simulink model "sim_new_traj_only_pos_ctrl"  (R2020a)
settings: Solver=ode4  StartTime=0.0  StopTime=30.0  FixedStep=0.01  RelTol=1e-3
values from neighbouring files (symbols this model uses):
  alfa_theta = 20    [init_new_traj_only_pos_ctrl.m]
  alfa_theta_obs = 100    [init_new_traj_only_pos_ctrl.m]
  beta1 = 1.2    [init_new_traj_only_pos_ctrl.m]
  beta2 = 0.8    [init_new_traj_only_pos_ctrl.m]
  c1_diff_sigma_bar_v = diag([25; 30; 20])    [init_new_traj_only_pos_ctrl.m]
  c1v = diag([5.8; 6.5; 6.5])    [init_new_traj_only_pos_ctrl.m]
  c2_diff_sigma_bar_v = diag([50; 50; 10])    [init_new_traj_only_pos_ctrl.m]
  c2v = diag([5.8; 6.5; 6.5])    [init_new_traj_only_pos_ctrl.m]
  c3_diff_sigma_bar_v = diag([15; 15; 10])    [init_new_traj_only_pos_ctrl.m]
  c3v = diag([4.8; 6.4; 6.0])    [init_new_traj_only_pos_ctrl.m]
  delta_p_i_0 = zeros(3, NF)    [init_new_traj_only_pos_ctrl.m]
  delta_v_i_0 = zeros(3, NF)    [init_new_traj_only_pos_ctrl.m]
  dp_aa_t = 0.2 * ones(3, 5) + ( 1.0 - 0.2 ) * rand(3, 5)    [init_new_traj_only_pos_ctrl.m]
  dp_ff_t = [ 0.4 * ones(1, 5) + ( 1.0 - 0.4 ) * rand(1, 5);                      0.4 * ones(1, 5) + ( 1.0 - 0.4 ) * rand(1, 5);                      0.2 * ones(1, 5) + ( 0.6 - 0.2 ) * rand(1, 5) ]    [init_new_traj_only_pos_ctrl.m]
  dp_phi_t = ( - pi / 2 ) * ones(3, 5) + ( pi / 2 - ( - pi / 2 ) ) * rand(3, 5)    [init_new_traj_only_pos_ctrl.m]
  etai_0 = zeros(3,5)    [init_new_traj_only_pos_ctrl.m]
  kai_1_t = 0.02    [init_new_traj_only_pos_ctrl.m]
  kai_3_t = 0.1    [init_new_traj_only_pos_ctrl.m]
  kai_chi_1 = diag([6; 6; 6])    [init_new_traj_only_pos_ctrl.m]
  kai_chi_2 = diag([6; 6; 6])    [init_new_traj_only_pos_ctrl.m]
  kai_u_1 = diag([8; 8; 8])    [init_new_traj_only_pos_ctrl.m]
  kai_u_2 = diag([8; 8; 8])    [init_new_traj_only_pos_ctrl.m]
  ksii_0 = zeros(3,5)    [init_new_traj_only_pos_ctrl.m]
  l1v = diag([20; 20; 20])    [init_new_traj_only_pos_ctrl.m]
  l2v = diag([30; 30; 30])    [init_new_traj_only_pos_ctrl.m]
  Lamd_diff_sigma_bar_v = 0.5    [init_new_traj_only_pos_ctrl.m]
  mass_i = zeros(1,NF)    [init_new_traj_only_pos_ctrl.m]
  Mii = diag([1;0;0;0;1])    [init_new_traj_only_pos_ctrl.m]
  pos0 = zeros(3, 1)    [init_new_traj_only_pos_ctrl.m]
  PZ0 = P0(3)    [init_new_traj_only_pos_ctrl.m]
  PZ1 = 10    [init_new_traj_only_pos_ctrl.m]
  Qci_init = repmat([1;0;0;0],1,NF)    [init_new_traj_only_pos_ctrl.m]
  R0 = 4    [init_new_traj_only_pos_ctrl.m]
  R1 = 8    [init_new_traj_only_pos_ctrl.m]
  Rx2 = 10    [init_new_traj_only_pos_ctrl.m]
  Ry2 = 6    [init_new_traj_only_pos_ctrl.m]
  Rz2 = 4    [init_new_traj_only_pos_ctrl.m]
  T0 = 0    [init_new_traj_only_pos_ctrl.m]
  T1 = tseq1    (= 10)    [init_new_traj_only_pos_ctrl.m]
  T12 = tseq1 + tseq12    (= 20)    [init_new_traj_only_pos_ctrl.m]
  T2 = tseq1 + tseq12 + tseq2    (= 30)    [init_new_traj_only_pos_ctrl.m]
  theta0 = ( 2 / 5 ) * pi    (= 1.25663706144)    [init_new_traj_only_pos_ctrl.m]
  vel0 = zeros(3, 1)    [init_new_traj_only_pos_ctrl.m]
  Wij = [0,0,1,0,0;              0,0,1,1,0;              1,0,0,0,1;              0,1,1,0,0;              0,0,1,0,0]    [init_new_traj_only_pos_ctrl.m]
  X1 = 8    [init_new_traj_only_pos_ctrl.m]
  X2 = 2    [init_new_traj_only_pos_ctrl.m]
  X3 = 3    [init_new_traj_only_pos_ctrl.m]
  Y1 = 10    [init_new_traj_only_pos_ctrl.m]
  Y2 = 2    [init_new_traj_only_pos_ctrl.m]
  Y3 = 4    [init_new_traj_only_pos_ctrl.m]
  Z1 = 4    [init_new_traj_only_pos_ctrl.m]
  Z2 = -6    [init_new_traj_only_pos_ctrl.m]
  Z3 = 2    [init_new_traj_only_pos_ctrl.m]
  zeta_diff_sigma_bar_v = 0.08    [init_new_traj_only_pos_ctrl.m]
undefined symbols (not defined in the file or in its folder): cal_frac_squ, p_alfav1, p_alfav2, p_beta1, p_beta2, p_dbeta1, p_dbeta2, p_gamma1_pos, p_gamma1_vel, p_gamma2_pos, p_gamma2_vel, q_alfav1, q_alfav2, q_beta1, q_beta2, q_dbeta1, q_dbeta2, q_gamma1_pos, q_gamma1_vel, q_gamma2_pos, q_gamma2_vel
(part 4 of 5)

== matlab function sim_new_traj_only_pos_ctrl/set desire formation configuration ==
  data: X1 input; X2 input; X3 input; Y1 input; Y2 input; Y3 input; Z1 input; Z2 input; Z3 input; theta0 input; kai_1_t input; kai_3_t input; T1 input; T12 input; t input; delta_ksi_vec output; delta_eta_vec output
function [delta_ksi_vec, delta_eta_vec] = fcn(X1, X2, X3, Y1, Y2, Y3, Z1, Z2, Z3, theta0, ...
                                                                                    kai_1_t, kai_3_t, T1, T12, t)
%%%% 计算跟随者期望速度分布式观测器误差
delta_ksi_vec = zeros(3, 5);
delta_eta_vec = zeros(3, 5);
if t <= ( T1 + 1e-04 )
    exp_tmp = exp( -kai_1_t * t );
    delta_ksi_vec(:, 1) = [ X1 * cos( theta0 ) - X2 * exp_tmp; ...
                                            Y1 * sin( theta0 ) - Y2 * exp_tmp; ...
                                            Z1 - Z2 * exp_tmp ];
    delta_ksi_vec(:, 2) = [ - X1 * cos( theta0 ) + X2 * exp_tmp; ...
                                            Y1 * sin( theta0 ) - Y2 * exp_tmp; ...
                                            Z1 + Z2 * exp_tmp ];
    delta_ksi_vec(:, 3) = [ X1 - X2 * exp_tmp; ...
                                            Y2 * exp_tmp; ...
                                            ( 3 / 8 ) * Z1 + Z2 * exp_tmp ];
    delta_ksi_vec(:, 4) = [ - X1 * cos( theta0 ) + X2 * exp_tmp; ...
                                            - Y1 * sin( theta0 ) + Y2 * exp_tmp; ...
                                            Z1 + Z2 * exp_tmp ];
    delta_ksi_vec(:, 5) = [ X1 * cos( theta0 ) - X2 * exp_tmp; ...
                                            - Y1 * sin( theta0 ) + Y2 * exp_tmp; ...
                                            Z1 - Z2 * exp_tmp ];
    delta_eta_vec(:, 1) = [ kai_1_t * X2 * exp_tmp; kai_1_t * Y2 * exp_tmp; kai_1_t * Z2 * exp_tmp ];
    delta_eta_vec(:, 2) = [ - kai_1_t * X2 * exp_tmp; kai_1_t * Y2 * exp_tmp; - kai_1_t * Z2 * exp_tmp ];
    delta_eta_vec(:, 3) = [ kai_1_t * X2 * exp_tmp; - kai_1_t * Y2 * exp_tmp; - kai_1_t * Z2 * exp_tmp ];
    delta_eta_vec(:, 4) = [ - kai_1_t * X2 * exp_tmp; - kai_1_t * Y2 * exp_tmp; - kai_1_t * Z2 * exp_tmp ];
    delta_eta_vec(:, 5) = [ kai_1_t * X2 * exp_tmp; - kai_1_t * Y2 * exp_tmp; kai_1_t * Z2 * exp_tmp ];
elseif t <= ( T12 + 1e-04 )
    delta_ksi_vec(:, 1) = [ X1 * cos( theta0 ) - X2; Y1 * sin( theta0 ) - Y2; Z1 - Z2 ];
    delta_ksi_vec(:, 2) = [ - X1 * cos( theta0 ) + X2; Y1 * sin( theta0 ) - Y2; Z1 + Z2 ];
    delta_ksi_vec(:, 3) = [ X1 - X2; 0; ( 3 / 8 ) * Z1 + Z2 ];
    delta_ksi_vec(:, 4) = [ - X1 * cos( theta0 ) + X2; - Y1 * sin( theta0 ) + Y2; Z1 + Z2 ];
    delta_ksi_vec(:, 5) = [ X1 * cos( theta0 ) - X2; - Y1 * sin( theta0 ) + Y2; Z1 - Z2 ];
else
    exp_tmp = 1 / ( 1 + exp( - kai_3_t * ( t - T12 - 5 ) ) );
    tmp_2 = exp( - kai_3_t * ( t - T12 - 5 ) ) / ( ( 1 + exp( - kai_3_t * ( t - T12 - 5 ) ) ) ^ 2 );
    delta_ksi_vec(:, 1) = [ X1 * cos( theta0 ) - X2 + X3 * exp_tmp; ...
                                            Y1 * sin( theta0 ) - Y2 + Y3 * exp_tmp; ...
                                            Z1 - Z2 + Z3 * exp_tmp ];
    delta_ksi_vec(:, 2) = [ - X1 * cos( theta0 ) + X2 - X3 * exp_tmp; ...
                                            Y1 * sin( theta0 ) - Y2 + Y3 * exp_tmp; ...
                                            Z1 + Z2 - Z3 * exp_tmp ];
    delta_ksi_vec(:, 3) = [ X1 - X2 + X3 * exp_tmp; ...
                                            - Y3 * exp_tmp; ...
                                            ( 3 / 8 ) * Z1 + Z2 - Z3 * exp_tmp ];
    delta_ksi_vec(:, 4) = [ - X1 * cos( theta0 ) + X2 - X3 * exp_tmp; ...
                                            - Y1 * sin( theta0 ) + Y2 - Y3 * exp_tmp; ...
                                            Z1 + Z2 - Z3 * exp_tmp ];
    delta_ksi_vec(:, 5) = [ X1 * cos( theta0 ) - X2 + X3 * exp_tmp; ...
                                            - Y1 * sin( theta0 ) + Y2 - Y3 * exp_tmp; ...
                                            Z1 - Z2 + Z3 * exp_tmp ];
    delta_eta_vec(:, 1) = [ kai_3_t * X3 * tmp_2; kai_3_t * Y3 * tmp_2; kai_3_t * Z3 * tmp_2 ];
    delta_eta_vec(:, 2) = [ - kai_3_t * X3 * tmp_2; kai_3_t * Y3 * tmp_2; kai_3_t * Z3 * tmp_2 ];
    delta_eta_vec(:, 3) = [ kai_3_t * X3 * tmp_2; - kai_3_t * Y3 * tmp_2; - kai_3_t * Z3 * tmp_2 ];
    delta_eta_vec(:, 4) = [ - kai_3_t * X3 * tmp_2; - kai_3_t * Y3 * tmp_2; - kai_3_t * Z3 * tmp_2 ];
    delta_eta_vec(:, 5) = [ kai_3_t * X3 * tmp_2; kai_3_t * Y3 * tmp_2; - kai_3_t * Z3 * tmp_2 ];
end

== matlab function sim_new_traj_only_pos_ctrl/choose dp_tilt_5 ==
  data: x input; y output
function y = fcn(x)
iiuav = 5;
y = x(:,iiuav);

== matlab function sim_new_traj_only_pos_ctrl/choose sigma_bar_v_tilt_5 ==
  data: x input; y output
function y = fcn(x)
iiuav = 5;
y = x(:,iiuav);

== matlab function sim_new_traj_only_pos_ctrl/choose sigma_bar_v_tilt_1 ==
  data: x input; y output
function y = fcn(x)
iiuav = 1;
y = x(:,iiuav);

== matlab function sim_new_traj_only_pos_ctrl/choose sigma_bar_v_tilt_2 ==
  data: x input; y output
function y = fcn(x)
iiuav = 2;
y = x(:,iiuav);

== matlab function sim_new_traj_only_pos_ctrl/choose sigma_bar_v_tilt_3 ==
  data: x input; y output
function y = fcn(x)
iiuav = 3;
y = x(:,iiuav);

== matlab function sim_new_traj_only_pos_ctrl/choose sigma_bar_v_tilt_4 ==
  data: x input; y output
function y = fcn(x)
iiuav = 4;
y = x(:,iiuav);

== matlab function sim_new_traj_only_pos_ctrl/choose phi_5 ==
  data: x input; y output
function y = fcn(x)
iiuav = 5;
y = x(:,iiuav);

== matlab function sim_new_traj_only_pos_ctrl/choose phi_1 ==
  data: x input; y output
function y = fcn(x)
iiuav = 1;
y = x(:,iiuav);

== matlab function sim_new_traj_only_pos_ctrl/choose phi_2 ==
  data: x input; y output
function y = fcn(x)
iiuav = 2;
y = x(:,iiuav);

== matlab function sim_new_traj_only_pos_ctrl/choose phi_3 ==
  data: x input; y output
function y = fcn(x)
iiuav = 3;
y = x(:,iiuav);

== matlab function sim_new_traj_only_pos_ctrl/choose phi_4 ==
  data: x input; y output
function y = fcn(x)
iiuav = 4;
y = x(:,iiuav);

== matlab function sim_new_traj_only_pos_ctrl/choose err_eta_1 ==
  data: x input; y output
function y = fcn(x)
iiuav = 1;
y = x(:,iiuav);

== matlab function sim_new_traj_only_pos_ctrl/choose chi_1 ==
  data: x input; y output
function y = fcn(x)
iiuav = 1;
y = x(:,iiuav);

== matlab function sim_new_traj_only_pos_ctrl/choose chi_2 ==
  data: x input; y output
function y = fcn(x)
iiuav = 2;
y = x(:,iiuav);

== matlab function sim_new_traj_only_pos_ctrl/choose err_eta_2 ==
  data: x input; y output
function y = fcn(x)
iiuav = 2;
y = x(:,iiuav);

== matlab function sim_new_traj_only_pos_ctrl/choose chi_3 ==
  data: x input; y output
function y = fcn(x)
iiuav = 3;
y = x(:,iiuav);

== matlab function sim_new_traj_only_pos_ctrl/choose err_eta_3 ==
  data: x input; y output
function y = fcn(x)
iiuav = 3;
y = x(:,iiuav);

== matlab function sim_new_traj_only_pos_ctrl/choose chi_4 ==
  data: x input; y output
function y = fcn(x)
iiuav = 4;
y = x(:,iiuav);

== matlab function sim_new_traj_only_pos_ctrl/choose err_eta_4 ==
  data: x input; y output
function y = fcn(x)
iiuav = 4;
y = x(:,iiuav);

== matlab function sim_new_traj_only_pos_ctrl/choose chi_5 ==
  data: x input; y output
function y = fcn(x)
iiuav = 5;
y = x(:,iiuav);

== matlab function sim_new_traj_only_pos_ctrl/choose err_eta_5 ==
  data: x input; y output
function y = fcn(x)
iiuav = 5;
y = x(:,iiuav);

== matlab function sim_new_traj_only_pos_ctrl/choose sigma_bar_v_hat_5 ==
  data: x input; y output
function y = fcn(x)
iiuav = 5;
y = x(:,iiuav);

== matlab function sim_new_traj_only_pos_ctrl/choose sigma_bar_v_hat_1 ==
  data: x input; y output
function y = fcn(x)
iiuav = 1;
y = x(:,iiuav);

== matlab function sim_new_traj_only_pos_ctrl/choose sigma_bar_v_hat_2 ==
  data: x input; y output
function y = fcn(x)
iiuav = 2;
y = x(:,iiuav);

== matlab function sim_new_traj_only_pos_ctrl/choose sigma_bar_v_hat_3 ==
  data: x input; y output
function y = fcn(x)
iiuav = 3;
y = x(:,iiuav);

== matlab function sim_new_traj_only_pos_ctrl/choose sigma_bar_v_hat_4 ==
  data: x input; y output
function y = fcn(x)
iiuav = 4;
y = x(:,iiuav);

== matlab function sim_new_traj_only_pos_ctrl/choose sigma_bar_v_5 ==
  data: x input; y output
function y = fcn(x)
iiuav = 5;
y = x(:,iiuav);

== matlab function sim_new_traj_only_pos_ctrl/choose sigma_bar_v_1 ==
  data: x input; y output
function y = fcn(x)
iiuav = 1;
y = x(:,iiuav);

== matlab function sim_new_traj_only_pos_ctrl/choose sigma_bar_v_2 ==
  data: x input; y output
function y = fcn(x)
iiuav = 2;
y = x(:,iiuav);

== matlab function sim_new_traj_only_pos_ctrl/choose sigma_bar_v_3 ==
  data: x input; y output
function y = fcn(x)
iiuav = 3;
y = x(:,iiuav);

== matlab function sim_new_traj_only_pos_ctrl/choose sigma_bar_v_4 ==
  data: x input; y output
function y = fcn(x)
iiuav = 4;
y = x(:,iiuav);

== matlab function sim_new_traj_only_pos_ctrl/cal formation tracking position and velocity errors ==
  data: ksi_i_vec input; err_ksi_vec output; ksi_d_est_vec input; eta_i_vec input; eta_d_est_vec input; err_eta_vec output
function [err_ksi_vec, err_eta_vec] = fcn(ksi_i_vec, ksi_d_est_vec, eta_i_vec, eta_d_est_vec)
%%%% 计算编队跟踪误差
err_ksi_vec = zeros(3,5);
err_eta_vec = zeros(3,5);
for iiuav = 1:5
    err_ksi_vec(:,iiuav) = ksi_i_vec(:,iiuav) - ksi_d_est_vec(:,iiuav);
    err_eta_vec(:,iiuav) = eta_i_vec(:,iiuav) - eta_d_est_vec(:,iiuav);
end

== matlab function sim_new_traj_only_pos_ctrl/choose dp_5 ==
  data: x input; y output
function y = fcn(x)
iiuav = 5;
y = x(:,iiuav);

== matlab function sim_new_traj_only_pos_ctrl/choose dp_1 ==
  data: x input; y output
function y = fcn(x)
iiuav = 1;
y = x(:,iiuav);

== matlab function sim_new_traj_only_pos_ctrl/choose dp_2 ==
  data: x input; y output
function y = fcn(x)
iiuav = 2;
y = x(:,iiuav);

== matlab function sim_new_traj_only_pos_ctrl/choose dp_3 ==
  data: x input; y output
function y = fcn(x)
iiuav = 3;
y = x(:,iiuav);

== matlab function sim_new_traj_only_pos_ctrl/choose dp_4 ==
  data: x input; y output
function y = fcn(x)
iiuav = 4;
y = x(:,iiuav);

== matlab function sim_new_traj_only_pos_ctrl/choose dp_hat_5 ==
  data: x input; y output
function y = fcn(x)
iiuav = 5;
y = x(:,iiuav);

== matlab function sim_new_traj_only_pos_ctrl/choose dp_hat_1 ==
  data: x input; y output
function y = fcn(x)
iiuav = 1;
y = x(:,iiuav);

== matlab function sim_new_traj_only_pos_ctrl/choose dp_hat_2 ==
  data: x input; y output
function y = fcn(x)
iiuav = 2;
y = x(:,iiuav);

== matlab function sim_new_traj_only_pos_ctrl/choose dp_hat_3 ==
  data: x input; y output
function y = fcn(x)
iiuav = 3;
y = x(:,iiuav);

== matlab function sim_new_traj_only_pos_ctrl/choose dp_hat_4 ==
  data: x input; y output
function y = fcn(x)
iiuav = 4;
y = x(:,iiuav);

== matlab function sim_new_traj_only_pos_ctrl/cal abs 41 ==
  data: x input; y output
function y = fcn(x)
y = abs(x(:));

== matlab function sim_new_traj_only_pos_ctrl/cal abs 42 ==
  data: x input; y output
function y = fcn(x)
y = abs(x(:));

== matlab function sim_new_traj_only_pos_ctrl/cal abs 43 ==
  data: x input; y output
function y = fcn(x)
y = abs(x(:));

== matlab function sim_new_traj_only_pos_ctrl/cal abs 44 ==
  data: x input; y output
function y = fcn(x)
y = abs(x(:));

== matlab function sim_new_traj_only_pos_ctrl/cal abs 45 ==
  data: x input; y output
function y = fcn(x)
y = abs(x(:));

== matlab function sim_new_traj_only_pos_ctrl/cal abs 46 ==
  data: x input; y output
function y = fcn(x)
y = abs(x(:));

== matlab function sim_new_traj_only_pos_ctrl/cal abs 1 ==
  data: x input; y output
function y = fcn(x)
y = abs(x(:));

== matlab function sim_new_traj_only_pos_ctrl/cal abs 47 ==
  data: x input; y output
function y = fcn(x)
y = abs(x(:));

== matlab function sim_new_traj_only_pos_ctrl/cal abs 48 ==
  data: x input; y output
function y = fcn(x)
y = abs(x(:));

== matlab function sim_new_traj_only_pos_ctrl/cal abs 49 ==
  data: x input; y output
function y = fcn(x)
y = abs(x(:));

== matlab function sim_new_traj_only_pos_ctrl/cal abs 50 ==
  data: x input; y output
function y = fcn(x)
y = abs(x(:));

== matlab function sim_new_traj_only_pos_ctrl/cal abs 51 ==
  data: x input; y output
function y = fcn(x)
y = abs(x(:));

== matlab function sim_new_traj_only_pos_ctrl/cal abs 52 ==
  data: x input; y output
function y = fcn(x)
y = abs(x(:));

== matlab function sim_new_traj_only_pos_ctrl/cal abs 53 ==
  data: x input; y output
function y = fcn(x)
y = abs(x(:));

== matlab function sim_new_traj_only_pos_ctrl/cal abs 54 ==
  data: x input; y output
function y = fcn(x)
y = abs(x(:));

== matlab function sim_new_traj_only_pos_ctrl/cal abs 55 ==
  data: x input; y output
function y = fcn(x)
y = abs(x(:));

== matlab function sim_new_traj_only_pos_ctrl/cal abs 56 ==
  data: x input; y output
function y = fcn(x)
y = abs(x(:));

== matlab function sim_new_traj_only_pos_ctrl/choose ksi_est_err 2 ==
  data: x input; y output
function y = fcn(x)
iiuav = 1;
y = x(:,iiuav);

== matlab function sim_new_traj_only_pos_ctrl/cal abs 57 ==
  data: x input; y output
function y = fcn(x)
y = abs(x(:));

== matlab function sim_new_traj_only_pos_ctrl/cal abs 58 ==
  data: x input; y output
function y = fcn(x)
y = abs(x(:));

== matlab function sim_new_traj_only_pos_ctrl/cal abs 59 ==
  data: x input; y output
function y = fcn(x)
y = abs(x(:));

== matlab function sim_new_traj_only_pos_ctrl/cal abs 60 ==
  data: x input; y output
function y = fcn(x)
y = abs(x(:));

== matlab function sim_new_traj_only_pos_ctrl/cal lumped observation error agent 1 ==
  data: wij input; w0 input; ksi_d_est_vec input; ksi0 input; delta_ksi_vec input; eta_d_est_vec input; ksi_est_err_tilt_1 output; eta0 input; delta_eta_vec input; eta_est_err_tilt_1 output
function [ksi_est_err_tilt_1, eta_est_err_tilt_1]  = fcn(wij, w0, ksi_d_est_vec, ksi0, delta_ksi_vec, eta_d_est_vec, eta0, delta_eta_vec)
%%%% 计算跟随者期望速度分布式观测器误差
iiuav = 1;
ksi_est_err_tilt_1 = w0(iiuav, iiuav) * (ksi_d_est_vec(:,iiuav) - ksi0(:) - delta_ksi_vec(:,iiuav));
eta_est_err_tilt_1 = w0(iiuav, iiuav) * (eta_d_est_vec(:,iiuav) - eta0(:) - delta_eta_vec(:,iiuav));
for jjuav = 1:5
    ksi_est_err_tilt_1 = ksi_est_err_tilt_1 + ...
                                        wij(iiuav, jjuav) * ((ksi_d_est_vec(:,iiuav) - delta_ksi_vec(:,iiuav)) - (ksi_d_est_vec(:,jjuav) - delta_ksi_vec(:,jjuav)));
    eta_est_err_tilt_1 = eta_est_err_tilt_1 + ...
                                        wij(iiuav, jjuav) * ((eta_d_est_vec(:,iiuav) - delta_eta_vec(:,iiuav)) - (eta_d_est_vec(:,jjuav) - delta_eta_vec(:,jjuav)));
end

== matlab function sim_new_traj_only_pos_ctrl/cal lumped observation error agent 2 ==
  data: wij input; w0 input; ksi_d_est_vec input; ksi0 input; delta_ksi_vec input; eta_d_est_vec input; ksi_est_err_tilt_2 output; eta0 input; delta_eta_vec input; eta_est_err_tilt_2 output
function [ksi_est_err_tilt_2, eta_est_err_tilt_2]  = fcn(wij, w0, ksi_d_est_vec, ksi0, delta_ksi_vec, eta_d_est_vec, eta0, delta_eta_vec)
%%%% 计算跟随者期望速度分布式观测器误差
iiuav = 2;
ksi_est_err_tilt_2 = w0(iiuav, iiuav) * (ksi_d_est_vec(:,iiuav) - ksi0(:) - delta_ksi_vec(:,iiuav));
eta_est_err_tilt_2 = w0(iiuav, iiuav) * (eta_d_est_vec(:,iiuav) - eta0(:) - delta_eta_vec(:,iiuav));
for jjuav = 1:5
    ksi_est_err_tilt_2 = ksi_est_err_tilt_2 + ...
                                        wij(iiuav, jjuav) * ((ksi_d_est_vec(:,iiuav) - delta_ksi_vec(:,iiuav)) - (ksi_d_est_vec(:,jjuav) - delta_ksi_vec(:,jjuav)));
    eta_est_err_tilt_2 = eta_est_err_tilt_2 + ...
                                        wij(iiuav, jjuav) * ((eta_d_est_vec(:,iiuav) - delta_eta_vec(:,iiuav)) - (eta_d_est_vec(:,jjuav) - delta_eta_vec(:,jjuav)));
end

== matlab function sim_new_traj_only_pos_ctrl/cal lumped observation error agent 3 ==
  data: wij input; w0 input; ksi_d_est_vec input; ksi0 input; delta_ksi_vec input; eta_d_est_vec input; ksi_est_err_tilt_3 output; eta0 input; delta_eta_vec input; eta_est_err_tilt_3 output
function [ksi_est_err_tilt_3, eta_est_err_tilt_3]  = fcn(wij, w0, ksi_d_est_vec, ksi0, delta_ksi_vec, eta_d_est_vec, eta0, delta_eta_vec)
%%%% 计算跟随者期望速度分布式观测器误差
iiuav = 3;
ksi_est_err_tilt_3 = w0(iiuav, iiuav) * (ksi_d_est_vec(:,iiuav) - ksi0(:) - delta_ksi_vec(:,iiuav));
eta_est_err_tilt_3 = w0(iiuav, iiuav) * (eta_d_est_vec(:,iiuav) - eta0(:) - delta_eta_vec(:,iiuav));
for jjuav = 1:5
    ksi_est_err_tilt_3 = ksi_est_err_tilt_3 + ...
                                        wij(iiuav, jjuav) * ((ksi_d_est_vec(:,iiuav) - delta_ksi_vec(:,iiuav)) - (ksi_d_est_vec(:,jjuav) - delta_ksi_vec(:,jjuav)));
    eta_est_err_tilt_3 = eta_est_err_tilt_3 + ...
                                        wij(iiuav, jjuav) * ((eta_d_est_vec(:,iiuav) - delta_eta_vec(:,iiuav)) - (eta_d_est_vec(:,jjuav) - delta_eta_vec(:,jjuav)));
end

== matlab function sim_new_traj_only_pos_ctrl/cal abs 6 ==
  data: x input; y output
function y = fcn(x)
y = abs(x(:));

== matlab function sim_new_traj_only_pos_ctrl/cal lumped observation error agent 4 ==
  data: wij input; w0 input; ksi_d_est_vec input; ksi0 input; delta_ksi_vec input; eta_d_est_vec input; ksi_est_err_tilt_4 output; eta0 input; delta_eta_vec input; eta_est_err_tilt_4 output
function [ksi_est_err_tilt_4, eta_est_err_tilt_4]  = fcn(wij, w0, ksi_d_est_vec, ksi0, delta_ksi_vec, eta_d_est_vec, eta0, delta_eta_vec)
%%%% 计算跟随者期望速度分布式观测器误差
iiuav = 4;
ksi_est_err_tilt_4 = w0(iiuav, iiuav) * (ksi_d_est_vec(:,iiuav) - ksi0(:) - delta_ksi_vec(:,iiuav));
eta_est_err_tilt_4 = w0(iiuav, iiuav) * (eta_d_est_vec(:,iiuav) - eta0(:) - delta_eta_vec(:,iiuav));
for jjuav = 1:5
    ksi_est_err_tilt_4 = ksi_est_err_tilt_4 + ...
                                        wij(iiuav, jjuav) * ((ksi_d_est_vec(:,iiuav) - delta_ksi_vec(:,iiuav)) - (ksi_d_est_vec(:,jjuav) - delta_ksi_vec(:,jjuav)));
    eta_est_err_tilt_4 = eta_est_err_tilt_4 + ...
                                        wij(iiuav, jjuav) * ((eta_d_est_vec(:,iiuav) - delta_eta_vec(:,iiuav)) - (eta_d_est_vec(:,jjuav) - delta_eta_vec(:,jjuav)));
end

== matlab function sim_new_traj_only_pos_ctrl/cal lumped observation error agent 5 ==
  data: wij input; w0 input; ksi_d_est_vec input; ksi0 input; delta_ksi_vec input; eta_d_est_vec input; ksi_est_err_tilt_5 output; eta0 input; delta_eta_vec input; eta_est_err_tilt_5 output
function [ksi_est_err_tilt_5, eta_est_err_tilt_5]  = fcn(wij, w0, ksi_d_est_vec, ksi0, delta_ksi_vec, eta_d_est_vec, eta0, delta_eta_vec)
%%%% 计算跟随者期望速度分布式观测器误差
iiuav = 5;
ksi_est_err_tilt_5 = w0(iiuav, iiuav) * (ksi_d_est_vec(:,iiuav) - ksi0(:) - delta_ksi_vec(:,iiuav));
eta_est_err_tilt_5 = w0(iiuav, iiuav) * (eta_d_est_vec(:,iiuav) - eta0(:) - delta_eta_vec(:,iiuav));
for jjuav = 1:5
    ksi_est_err_tilt_5 = ksi_est_err_tilt_5 + ...
                                        wij(iiuav, jjuav) * ((ksi_d_est_vec(:,iiuav) - delta_ksi_vec(:,iiuav)) - (ksi_d_est_vec(:,jjuav) - delta_ksi_vec(:,jjuav)));
    eta_est_err_tilt_5 = eta_est_err_tilt_5 + ...
                                        wij(iiuav, jjuav) * ((eta_d_est_vec(:,iiuav) - delta_eta_vec(:,iiuav)) - (eta_d_est_vec(:,jjuav) - delta_eta_vec(:,jjuav)));
end

== matlab function sim_new_traj_only_pos_ctrl/cal position estimate error ==
  data: ksi_d_est_vec input; ksi_est_err output; ksi0 input; delta_ksi_vec input
function ksi_est_err  = fcn(ksi_d_est_vec, ksi0, delta_ksi_vec)
%%%% 计算跟随者期望位置分布式观测器误差
ksi_est_err = ksi_d_est_vec - repmat(ksi0, 1, 5) - delta_ksi_vec;

== matlab function sim_new_traj_only_pos_ctrl/cal theta_eta_est_err_tilt agent 1 ==
  data: alfa_theta input; eta_est_err_squ_1_node_1 input; theta_eta_est_err_tilt_1_1 output; eta_est_err_squ_2_node_1 input; eta_est_err_tilt_vec input; theta_eta_est_err_tilt_2_1 output
function [theta_eta_est_err_tilt_1_1, theta_eta_est_err_tilt_2_1] = fcn(alfa_theta, eta_est_err_squ_1_node_1, eta_est_err_squ_2_node_1, eta_est_err_tilt_vec)
%%%% 计算平滑递增函数
iiuav = 1;
theta_eta_est_err_tilt_1_1 = eta_est_err_squ_1_node_1(:) .* ( -1 + 2 ./ ( 1 + exp( -alfa_theta .* eta_est_err_tilt_vec(:,iiuav) ) ) );
theta_eta_est_err_tilt_2_1 = eta_est_err_squ_2_node_1(:) .* ( -1 + 2 ./ ( 1 + exp( -alfa_theta .* eta_est_err_tilt_vec(:,iiuav) ) ) );

== matlab function sim_new_traj_only_pos_ctrl/cal theta_eta_est_err_tilt agent 2 ==
  data: alfa_theta input; eta_est_err_squ_1_node_2 input; theta_eta_est_err_tilt_1_2 output; eta_est_err_squ_2_node_2 input; eta_est_err_tilt_vec input; theta_eta_est_err_tilt_2_2 output
function [theta_eta_est_err_tilt_1_2, theta_eta_est_err_tilt_2_2] = fcn(alfa_theta, eta_est_err_squ_1_node_2, eta_est_err_squ_2_node_2, eta_est_err_tilt_vec)
%%%% 计算平滑递增函数
iiuav = 2;
theta_eta_est_err_tilt_1_2 = eta_est_err_squ_1_node_2(:) .* ( -1 + 2 ./ ( 1 + exp( -alfa_theta .* eta_est_err_tilt_vec(:,iiuav) ) ) );
theta_eta_est_err_tilt_2_2 = eta_est_err_squ_2_node_2(:) .* ( -1 + 2 ./ ( 1 + exp( -alfa_theta .* eta_est_err_tilt_vec(:,iiuav) ) ) );

== matlab function sim_new_traj_only_pos_ctrl/cal theta_eta_est_err_tilt agent 3 ==
  data: alfa_theta input; eta_est_err_squ_1_node_3 input; theta_eta_est_err_tilt_1_3 output; eta_est_err_squ_2_node_3 input; eta_est_err_tilt_vec input; theta_eta_est_err_tilt_2_3 output
function [theta_eta_est_err_tilt_1_3, theta_eta_est_err_tilt_2_3] = fcn(alfa_theta, eta_est_err_squ_1_node_3, eta_est_err_squ_2_node_3, eta_est_err_tilt_vec)
%%%% 计算平滑递增函数
iiuav = 3;
theta_eta_est_err_tilt_1_3 = eta_est_err_squ_1_node_3(:) .* ( -1 + 2 ./ ( 1 + exp( -alfa_theta .* eta_est_err_tilt_vec(:,iiuav) ) ) );
theta_eta_est_err_tilt_2_3 = eta_est_err_squ_2_node_3(:) .* ( -1 + 2 ./ ( 1 + exp( -alfa_theta .* eta_est_err_tilt_vec(:,iiuav) ) ) );

== matlab function sim_new_traj_only_pos_ctrl/cal theta_err_ksi agent 3 ==
  data: alfa_theta input; err_ksi_squ_1_node_3 input; theta_err_ksi_1_3 output; err_ksi_squ_2_node_3 input; err_ksi_vec input; theta_err_ksi_2_3 output
function [theta_err_ksi_1_3, theta_err_ksi_2_3] = fcn(alfa_theta, err_ksi_squ_1_node_3, err_ksi_squ_2_node_3, err_ksi_vec)
%%%% 计算平滑递增函数
iiuav = 3;
theta_err_ksi_1_3 = err_ksi_squ_1_node_3(:) .* ( -1 + 2 ./ ( 1 + exp( -alfa_theta .* err_ksi_vec(:,iiuav) ) ) );
theta_err_ksi_2_3 = err_ksi_squ_2_node_3(:) .* ( -1 + 2 ./ ( 1 + exp( -alfa_theta .* err_ksi_vec(:,iiuav) ) ) );

== matlab function sim_new_traj_only_pos_ctrl/cal theta_eta_est_err_tilt agent 4 ==
  data: alfa_theta input; eta_est_err_squ_1_node_4 input; theta_eta_est_err_tilt_1_4 output; eta_est_err_squ_2_node_4 input; eta_est_err_tilt_vec input; theta_eta_est_err_tilt_2_4 output
function [theta_eta_est_err_tilt_1_4, theta_eta_est_err_tilt_2_4] = fcn(alfa_theta, eta_est_err_squ_1_node_4, eta_est_err_squ_2_node_4, eta_est_err_tilt_vec)
%%%% 计算平滑递增函数
iiuav = 4;
theta_eta_est_err_tilt_1_4 = eta_est_err_squ_1_node_4(:) .* ( -1 + 2 ./ ( 1 + exp( -alfa_theta .* eta_est_err_tilt_vec(:,iiuav) ) ) );
theta_eta_est_err_tilt_2_4 = eta_est_err_squ_2_node_4(:) .* ( -1 + 2 ./ ( 1 + exp( -alfa_theta .* eta_est_err_tilt_vec(:,iiuav) ) ) );

== matlab function sim_new_traj_only_pos_ctrl/cal theta_eta_est_err_tilt agent 5 ==
  data: alfa_theta input; eta_est_err_squ_1_node_5 input; theta_eta_est_err_tilt_1_5 output; eta_est_err_squ_2_node_5 input; eta_est_err_tilt_vec input; theta_eta_est_err_tilt_2_5 output
function [theta_eta_est_err_tilt_1_5, theta_eta_est_err_tilt_2_5] = fcn(alfa_theta, eta_est_err_squ_1_node_5, eta_est_err_squ_2_node_5, eta_est_err_tilt_vec)
%%%% 计算平滑递增函数
iiuav = 5;
theta_eta_est_err_tilt_1_5 = eta_est_err_squ_1_node_5(:) .* ( -1 + 2 ./ ( 1 + exp( -alfa_theta .* eta_est_err_tilt_vec(:,iiuav) ) ) );
theta_eta_est_err_tilt_2_5 = eta_est_err_squ_2_node_5(:) .* ( -1 + 2 ./ ( 1 + exp( -alfa_theta .* eta_est_err_tilt_vec(:,iiuav) ) ) );

== matlab function sim_new_traj_only_pos_ctrl/cal theta_ksi_est_err_tilt agent 1 ==
  data: alfa_theta input; ksi_est_err_squ_1_node_1 input; theta_ksi_est_err_tilt_1_1 output; ksi_est_err_squ_2_node_1 input; ksi_est_err_tilt_vec input; theta_ksi_est_err_tilt_2_1 output
function [theta_ksi_est_err_tilt_1_1, theta_ksi_est_err_tilt_2_1] = fcn(alfa_theta, ksi_est_err_squ_1_node_1, ksi_est_err_squ_2_node_1, ksi_est_err_tilt_vec)
%%%% 计算平滑递增函数
iiuav = 1;
theta_ksi_est_err_tilt_1_1 = ksi_est_err_squ_1_node_1(:) .* ( -1 + 2 ./ ( 1 + exp( -alfa_theta .* ksi_est_err_tilt_vec(:,iiuav) ) ) );
theta_ksi_est_err_tilt_2_1 = ksi_est_err_squ_2_node_1(:) .* ( -1 + 2 ./ ( 1 + exp( -alfa_theta .* ksi_est_err_tilt_vec(:,iiuav) ) ) );

== matlab function sim_new_traj_only_pos_ctrl/cal theta_ksi_est_err_tilt agent 2 ==
  data: alfa_theta input; ksi_est_err_squ_1_node_2 input; theta_ksi_est_err_tilt_1_2 output; ksi_est_err_squ_2_node_2 input; ksi_est_err_tilt_vec input; theta_ksi_est_err_tilt_2_2 output
function [theta_ksi_est_err_tilt_1_2, theta_ksi_est_err_tilt_2_2] = fcn(alfa_theta, ksi_est_err_squ_1_node_2, ksi_est_err_squ_2_node_2, ksi_est_err_tilt_vec)
%%%% 计算平滑递增函数
iiuav = 2;
theta_ksi_est_err_tilt_1_2 = ksi_est_err_squ_1_node_2(:) .* ( -1 + 2 ./ ( 1 + exp( -alfa_theta .* ksi_est_err_tilt_vec(:,iiuav) ) ) );
theta_ksi_est_err_tilt_2_2 = ksi_est_err_squ_2_node_2(:) .* ( -1 + 2 ./ ( 1 + exp( -alfa_theta .* ksi_est_err_tilt_vec(:,iiuav) ) ) );

== matlab function sim_new_traj_only_pos_ctrl/cal theta_ksi_est_err_tilt agent 3 ==
  data: alfa_theta input; ksi_est_err_squ_1_node_3 input; theta_ksi_est_err_tilt_1_3 output; ksi_est_err_squ_2_node_3 input; ksi_est_err_tilt_vec input; theta_ksi_est_err_tilt_2_3 output
function [theta_ksi_est_err_tilt_1_3, theta_ksi_est_err_tilt_2_3] = fcn(alfa_theta, ksi_est_err_squ_1_node_3, ksi_est_err_squ_2_node_3, ksi_est_err_tilt_vec)
%%%% 计算平滑递增函数
iiuav = 3;
theta_ksi_est_err_tilt_1_3 = ksi_est_err_squ_1_node_3(:) .* ( -1 + 2 ./ ( 1 + exp( -alfa_theta .* ksi_est_err_tilt_vec(:,iiuav) ) ) );
theta_ksi_est_err_tilt_2_3 = ksi_est_err_squ_2_node_3(:) .* ( -1 + 2 ./ ( 1 + exp( -alfa_theta .* ksi_est_err_tilt_vec(:,iiuav) ) ) );

== matlab function sim_new_traj_only_pos_ctrl/cal theta_ksi_est_err_tilt agent 4 ==
  data: alfa_theta input; ksi_est_err_squ_1_node_4 input; theta_ksi_est_err_tilt_1_4 output; ksi_est_err_squ_2_node_4 input; ksi_est_err_tilt_vec input; theta_ksi_est_err_tilt_2_4 output
function [theta_ksi_est_err_tilt_1_4, theta_ksi_est_err_tilt_2_4] = fcn(alfa_theta, ksi_est_err_squ_1_node_4, ksi_est_err_squ_2_node_4, ksi_est_err_tilt_vec)
%%%% 计算平滑递增函数
iiuav = 4;
theta_ksi_est_err_tilt_1_4 = ksi_est_err_squ_1_node_4(:) .* ( -1 + 2 ./ ( 1 + exp( -alfa_theta .* ksi_est_err_tilt_vec(:,iiuav) ) ) );
theta_ksi_est_err_tilt_2_4 = ksi_est_err_squ_2_node_4(:) .* ( -1 + 2 ./ ( 1 + exp( -alfa_theta .* ksi_est_err_tilt_vec(:,iiuav) ) ) );

== matlab function sim_new_traj_only_pos_ctrl/cal theta_ksi_est_err_tilt agent 5 ==
  data: alfa_theta input; ksi_est_err_squ_1_node_5 input; theta_ksi_est_err_tilt_1_5 output; ksi_est_err_squ_2_node_5 input; ksi_est_err_tilt_vec input; theta_ksi_est_err_tilt_2_5 output
function [theta_ksi_est_err_tilt_1_5, theta_ksi_est_err_tilt_2_5] = fcn(alfa_theta, ksi_est_err_squ_1_node_5, ksi_est_err_squ_2_node_5, ksi_est_err_tilt_vec)
%%%% 计算平滑递增函数
iiuav = 5;
theta_ksi_est_err_tilt_1_5 = ksi_est_err_squ_1_node_5(:) .* ( -1 + 2 ./ ( 1 + exp( -alfa_theta .* ksi_est_err_tilt_vec(:,iiuav) ) ) );
theta_ksi_est_err_tilt_2_5 = ksi_est_err_squ_2_node_5(:) .* ( -1 + 2 ./ ( 1 + exp( -alfa_theta .* ksi_est_err_tilt_vec(:,iiuav) ) ) );

== matlab function sim_new_traj_only_pos_ctrl/cal velocity estimate error ==
  data: eta_d_est_vec input; eta_est_err output; eta0 input; delta_eta_vec input
function eta_est_err  = fcn(eta_d_est_vec, eta0, delta_eta_vec)
%%%% 计算跟随者期望速度分布式观测器误差
eta_est_err = eta_d_est_vec - repmat(eta0, 1, 5) - delta_eta_vec;

== matlab function sim_new_traj_only_pos_ctrl/choose eta_est_err_tilt 1 ==
  data: x input; y output
function y = fcn(x)
iiuav = 1;
y = x(:,iiuav);

== matlab function sim_new_traj_only_pos_ctrl/choose eta_est_err_tilt 10 ==
  data: x input; y output
function y = fcn(x)
iiuav = 5;
y = x(:,iiuav);

== matlab function sim_new_traj_only_pos_ctrl/choose eta_est_err_tilt 11 ==
  data: x input; y output
function y = fcn(x)
iiuav = 1;
y = x(:,iiuav);

== matlab function sim_new_traj_only_pos_ctrl/choose ksi_est_err 5 ==
  data: x input; y output
function y = fcn(x)
iiuav = 3;
y = x(:,iiuav);

== matlab function sim_new_traj_only_pos_ctrl/choose eta_est_err_tilt 12 ==
  data: x input; y output
function y = fcn(x)
iiuav = 5;
y = x(:,iiuav);

== matlab function sim_new_traj_only_pos_ctrl/choose eta_est_err_tilt 13 ==
  data: x input; y output
function y = fcn(x)
iiuav = 1;
y = x(:,iiuav);

== matlab function sim_new_traj_only_pos_ctrl/choose eta_est_err_tilt 14 ==
  data: x input; y output
function y = fcn(x)
iiuav = 2;
y = x(:,iiuav);

== matlab function sim_new_traj_only_pos_ctrl/choose eta_est_err_tilt 15 ==
  data: x input; y output
function y = fcn(x)
iiuav = 2;
y = x(:,iiuav);

== matlab function sim_new_traj_only_pos_ctrl/choose eta_est_err_tilt 16 ==
  data: x input; y output
function y = fcn(x)
iiuav = 3;
y = x(:,iiuav);

== matlab function sim_new_traj_only_pos_ctrl/choose eta_est_err_tilt 17 ==
  data: x input; y output
function y = fcn(x)
iiuav = 3;
y = x(:,iiuav);

== matlab function sim_new_traj_only_pos_ctrl/choose eta_est_err_tilt 18 ==
  data: x input; y output
function y = fcn(x)
iiuav = 4;
y = x(:,iiuav);

== matlab function sim_new_traj_only_pos_ctrl/choose eta_est_err_tilt 19 ==
  data: x input; y output
function y = fcn(x)
iiuav = 4;
y = x(:,iiuav);

== matlab function sim_new_traj_only_pos_ctrl/choose eta_est_err_tilt 2 ==
  data: x input; y output
function y = fcn(x)
iiuav = 1;
y = x(:,iiuav);

== matlab function sim_new_traj_only_pos_ctrl/choose eta_est_err_tilt 20 ==
  data: x input; y output
function y = fcn(x)
iiuav = 5;
y = x(:,iiuav);

== matlab function sim_new_traj_only_pos_ctrl/choose ksi_est_err 6 ==
  data: x input; y output
function y = fcn(x)
iiuav = 3;
y = x(:,iiuav);

== matlab function sim_new_traj_only_pos_ctrl/choose eta_est_err_tilt 3 ==
  data: x input; y output
function y = fcn(x)
iiuav = 2;
y = x(:,iiuav);

== matlab function sim_new_traj_only_pos_ctrl/choose eta_est_err_tilt 4 ==
  data: x input; y output
function y = fcn(x)
iiuav = 2;
y = x(:,iiuav);

== matlab function sim_new_traj_only_pos_ctrl/choose eta_est_err_tilt 5 ==
  data: x input; y output
function y = fcn(x)
iiuav = 3;
y = x(:,iiuav);

== matlab function sim_new_traj_only_pos_ctrl/choose eta_est_err_tilt 6 ==
  data: x input; y output
function y = fcn(x)
iiuav = 3;
y = x(:,iiuav);

== matlab function sim_new_traj_only_pos_ctrl/choose eta_est_err_tilt 7 ==
  data: x input; y output
function y = fcn(x)
iiuav = 4;
y = x(:,iiuav);

== matlab function sim_new_traj_only_pos_ctrl/choose eta_est_err_tilt 8 ==
  data: x input; y output
function y = fcn(x)
iiuav = 4;
y = x(:,iiuav);

== matlab function sim_new_traj_only_pos_ctrl/choose eta_est_err_tilt 9 ==
  data: x input; y output
function y = fcn(x)
iiuav = 5;
y = x(:,iiuav);

== matlab function sim_new_traj_only_pos_ctrl/combine follower desire velocity estimaters ==
  data: eta_d_est_1 input; eta_d_est_vec output; eta_d_est_2 input; eta_d_est_3 input; eta_d_est_4 input; eta_d_est_5 input
function eta_d_est_vec = fcn(eta_d_est_1, eta_d_est_2, eta_d_est_3, eta_d_est_4, eta_d_est_5)
%%%% 合并领导者位置观测器输出结果
eta_d_est_vec = [eta_d_est_1(:), eta_d_est_2(:), eta_d_est_3(:), eta_d_est_4(:), eta_d_est_5(:)];

== matlab function sim_new_traj_only_pos_ctrl/combine leader position estimaters ==
  data: ksi_d_est_1 input; ksi_d_est_vec output; ksi_d_est_2 input; ksi_d_est_3 input; ksi_d_est_4 input; ksi_d_est_5 input
function ksi_d_est_vec  = fcn(ksi_d_est_1, ksi_d_est_2, ksi_d_est_3, ksi_d_est_4, ksi_d_est_5)
%%%% 合并领导者位置观测器输出结果
ksi_d_est_vec = [ksi_d_est_1(:), ksi_d_est_2(:), ksi_d_est_3(:), ksi_d_est_4(:), ksi_d_est_5(:)];

== matlab function sim_new_traj_only_pos_ctrl/trans to column4 ==
  data: x input; y output
function y = fcn(x)
y = x(:);

== matlab function sim_new_traj_only_pos_ctrl/combine lumped follower observation error  ==
  data: ksi_est_err_tilt_1 input; ksi_est_err_tilt_2 input; ksi_est_err_tilt_3 input; ksi_est_err_tilt_4 input; ksi_est_err_tilt_5 input; ksi_est_err_tilt_vec output; eta_est_err_tilt_1 input; eta_est_err_tilt_vec output; eta_est_err_tilt_2 input; eta_est_err_tilt_3 input; eta_est_err_tilt_4 input; eta_est_err_tilt_5 input
function [ksi_est_err_tilt_vec, eta_est_err_tilt_vec]  = fcn(ksi_est_err_tilt_1, ksi_est_err_tilt_2, ksi_est_err_tilt_3, ksi_est_err_tilt_4, ksi_est_err_tilt_5, ...
                                                                                                        eta_est_err_tilt_1, eta_est_err_tilt_2, eta_est_err_tilt_3, eta_est_err_tilt_4, eta_est_err_tilt_5)
%%%% 合并领导者位置观测器输出结果
ksi_est_err_tilt_vec = [ksi_est_err_tilt_1, ksi_est_err_tilt_2, ksi_est_err_tilt_3, ksi_est_err_tilt_4, ksi_est_err_tilt_5];
eta_est_err_tilt_vec = [eta_est_err_tilt_1, eta_est_err_tilt_2, eta_est_err_tilt_3, eta_est_err_tilt_4, eta_est_err_tilt_5];

== matlab function sim_new_traj_only_pos_ctrl/combine lumped follower position observation error ==
  data: theta_ksi_est_err_tilt_1_1 input; theta_ksi_est_err_tilt_1_2 input; theta_ksi_est_err_tilt_1_3 input; theta_ksi_est_err_tilt_1_4 input; theta_ksi_est_err_tilt_1_5 input; theta_ksi_est_err_tilt_1_vec output; theta_ksi_est_err_tilt_2_1 input; theta_ksi_est_err_tilt_2_vec output; theta_ksi_est_err_tilt_2_2 input; theta_ksi_est_err_tilt_2_3 input; theta_ksi_est_err_tilt_2_4 input; theta_ksi_est_err_tilt_2_5 input
function [theta_ksi_est_err_tilt_1_vec, theta_ksi_est_err_tilt_2_vec]  = fcn(theta_ksi_est_err_tilt_1_1, theta_ksi_est_err_tilt_1_2, theta_ksi_est_err_tilt_1_3, theta_ksi_est_err_tilt_1_4, theta_ksi_est_err_tilt_1_5, ...
                                                                                                                                    theta_ksi_est_err_tilt_2_1, theta_ksi_est_err_tilt_2_2, theta_ksi_est_err_tilt_2_3, theta_ksi_est_err_tilt_2_4, theta_ksi_est_err_tilt_2_5)
%%%% 合并领导者位置观测器输出结果
theta_ksi_est_err_tilt_1_vec = [theta_ksi_est_err_tilt_1_1(:), theta_ksi_est_err_tilt_1_2(:), theta_ksi_est_err_tilt_1_3(:), theta_ksi_est_err_tilt_1_4(:), theta_ksi_est_err_tilt_1_5(:)];
theta_ksi_est_err_tilt_2_vec = [theta_ksi_est_err_tilt_2_1(:), theta_ksi_est_err_tilt_2_2(:), theta_ksi_est_err_tilt_2_3(:), theta_ksi_est_err_tilt_2_4(:), theta_ksi_est_err_tilt_2_5(:)];

== matlab function sim_new_traj_only_pos_ctrl/combine lumped follower velocity observation error ==
  data: theta_eta_est_err_tilt_1_1 input; theta_eta_est_err_tilt_1_2 input; theta_eta_est_err_tilt_1_3 input; theta_eta_est_err_tilt_1_4 input; theta_eta_est_err_tilt_1_5 input; theta_eta_est_err_tilt_1_vec output; theta_eta_est_err_tilt_2_1 input; theta_eta_est_err_tilt_2_vec output; theta_eta_est_err_tilt_2_2 input; theta_eta_est_err_tilt_2_3 input; theta_eta_est_err_tilt_2_4 input; theta_eta_est_err_tilt_2_5 input
function [theta_eta_est_err_tilt_1_vec, theta_eta_est_err_tilt_2_vec]  = fcn(theta_eta_est_err_tilt_1_1, theta_eta_est_err_tilt_1_2, theta_eta_est_err_tilt_1_3, theta_eta_est_err_tilt_1_4, theta_eta_est_err_tilt_1_5, ...
                                                                                                                                    theta_eta_est_err_tilt_2_1, theta_eta_est_err_tilt_2_2, theta_eta_est_err_tilt_2_3, theta_eta_est_err_tilt_2_4, theta_eta_est_err_tilt_2_5)
%%%% 合并领导者位置观测器输出结果
theta_eta_est_err_tilt_1_vec = [theta_eta_est_err_tilt_1_1(:), theta_eta_est_err_tilt_1_2(:), theta_eta_est_err_tilt_1_3(:), theta_eta_est_err_tilt_1_4(:), theta_eta_est_err_tilt_1_5(:)];
theta_eta_est_err_tilt_2_vec = [theta_eta_est_err_tilt_2_1(:), theta_eta_est_err_tilt_2_2(:), theta_eta_est_err_tilt_2_3(:), theta_eta_est_err_tilt_2_4(:), theta_eta_est_err_tilt_2_5(:)];

== matlab function sim_new_traj_only_pos_ctrl/divide eta_est_err ==
  data: eta_est_err input; eta_est_err_1 output; eta_est_err_2 output; eta_est_err_3 output; eta_est_err_4 output; eta_est_err_5 output
function [eta_est_err_1, eta_est_err_2, eta_est_err_3, eta_est_err_4, eta_est_err_5]  = fcn(eta_est_err)
%%%% 计算跟随者期望位置分布式观测器误差
eta_est_err_1 = eta_est_err(:,1);
eta_est_err_2 = eta_est_err(:,2);
eta_est_err_3 = eta_est_err(:,3);
eta_est_err_4 = eta_est_err(:,4);
eta_est_err_5 = eta_est_err(:,5);

== matlab function sim_new_traj_only_pos_ctrl/divide ksi_est_err ==
  data: ksi_est_err input; ksi_est_err_1 output; ksi_est_err_2 output; ksi_est_err_3 output; ksi_est_err_4 output; ksi_est_err_5 output
function [ksi_est_err_1, ksi_est_err_2, ksi_est_err_3, ksi_est_err_4, ksi_est_err_5]  = fcn(ksi_est_err)
%%%% 计算跟随者期望位置分布式观测器误差
ksi_est_err_1 = ksi_est_err(:,1);
ksi_est_err_2 = ksi_est_err(:,2);
ksi_est_err_3 = ksi_est_err(:,3);
ksi_est_err_4 = ksi_est_err(:,4);
ksi_est_err_5 = ksi_est_err(:,5);

== matlab function sim_new_traj_only_pos_ctrl/trans to column5 ==
  data: x input; y output
function y = fcn(x)
y = x(:);

== matlab function sim_new_traj_only_pos_ctrl/fixed-time distributed follower desire position observer agent 1 ==
  data: l1p input; d_ksi_d_est_1 output; l2p input; eta_d_est_vec input; theta_ksi_est_err_tilt_1_vec input; theta_ksi_est_err_tilt_2_vec input
function d_ksi_d_est_1 = fcn(l1p, l2p, eta_d_est_vec, theta_ksi_est_err_tilt_1_vec, theta_ksi_est_err_tilt_2_vec)
%%%% 固定时间跟随者期望位置分布式观测器
iiuav = 1;
d_ksi_d_est_1 = eta_d_est_vec(:,iiuav) - l1p * theta_ksi_est_err_tilt_1_vec(:,iiuav) - l2p * theta_ksi_est_err_tilt_2_vec(:,iiuav);

== matlab function sim_new_traj_only_pos_ctrl/fixed-time distributed follower desire position observer agent 2 ==
  data: l1p input; d_ksi_d_est_2 output; l2p input; eta_d_est_vec input; theta_ksi_est_err_tilt_1_vec input; theta_ksi_est_err_tilt_2_vec input
function d_ksi_d_est_2 = fcn(l1p, l2p, eta_d_est_vec, theta_ksi_est_err_tilt_1_vec, theta_ksi_est_err_tilt_2_vec)
%%%% 固定时间跟随者期望位置分布式观测器
iiuav = 2;
d_ksi_d_est_2 = eta_d_est_vec(:,iiuav) - l1p * theta_ksi_est_err_tilt_1_vec(:,iiuav) - l2p * theta_ksi_est_err_tilt_2_vec(:,iiuav);

== matlab function sim_new_traj_only_pos_ctrl/fixed-time distributed follower desire position observer agent 3 ==
  data: l1p input; d_ksi_d_est_3 output; l2p input; eta_d_est_vec input; theta_ksi_est_err_tilt_1_vec input; theta_ksi_est_err_tilt_2_vec input
function d_ksi_d_est_3 = fcn(l1p, l2p, eta_d_est_vec, theta_ksi_est_err_tilt_1_vec, theta_ksi_est_err_tilt_2_vec)
%%%% 固定时间跟随者期望位置分布式观测器
iiuav = 3;
d_ksi_d_est_3 = eta_d_est_vec(:,iiuav) - l1p * theta_ksi_est_err_tilt_1_vec(:,iiuav) - l2p * theta_ksi_est_err_tilt_2_vec(:,iiuav);

== matlab function sim_new_traj_only_pos_ctrl/fixed-time distributed follower desire position observer agent 4 ==
  data: l1p input; d_ksi_d_est_4 output; l2p input; eta_d_est_vec input; theta_ksi_est_err_tilt_1_vec input; theta_ksi_est_err_tilt_2_vec input
function d_ksi_d_est_4 = fcn(l1p, l2p, eta_d_est_vec, theta_ksi_est_err_tilt_1_vec, theta_ksi_est_err_tilt_2_vec)
%%%% 固定时间跟随者期望位置分布式观测器
iiuav = 4;
d_ksi_d_est_4 = eta_d_est_vec(:,iiuav) - l1p * theta_ksi_est_err_tilt_1_vec(:,iiuav) - l2p * theta_ksi_est_err_tilt_2_vec(:,iiuav);

== matlab function sim_new_traj_only_pos_ctrl/fixed-time distributed follower desire position observer agent 5 ==
  data: l1p input; d_ksi_d_est_5 output; l2p input; eta_d_est_vec input; theta_ksi_est_err_tilt_1_vec input; theta_ksi_est_err_tilt_2_vec input
function d_ksi_d_est_5 = fcn(l1p, l2p, eta_d_est_vec, theta_ksi_est_err_tilt_1_vec, theta_ksi_est_err_tilt_2_vec)
%%%% 固定时间跟随者期望位置分布式观测器
iiuav = 5;
d_ksi_d_est_5 = eta_d_est_vec(:,iiuav) - l1p * theta_ksi_est_err_tilt_1_vec(:,iiuav) - l2p * theta_ksi_est_err_tilt_2_vec(:,iiuav);

== matlab function sim_new_traj_only_pos_ctrl/fixed-time distributed follower desire velocity observer agent 1 ==
  data: l1v input; d_eta_d_est_1 output; l2v input; theta_eta_est_err_tilt_1_vec input; theta_eta_est_err_tilt_2_vec input
function d_eta_d_est_1 = fcn(l1v, l2v, theta_eta_est_err_tilt_1_vec, theta_eta_est_err_tilt_2_vec)
%%%% 固定时间跟随者期望速度分布式观测器
iiuav = 1;
d_eta_d_est_1 = -l1v * theta_eta_est_err_tilt_1_vec(:,iiuav) - l2v * theta_eta_est_err_tilt_2_vec(:,iiuav);

== matlab function sim_new_traj_only_pos_ctrl/cal abs 7 ==
  data: x input; y output
function y = fcn(x)
y = abs(x(:));

== matlab function sim_new_traj_only_pos_ctrl/fixed-time distributed follower desire velocity observer agent 2 ==
  data: l1v input; d_eta_d_est_2 output; l2v input; theta_eta_est_err_tilt_1_vec input; theta_eta_est_err_tilt_2_vec input
function d_eta_d_est_2 = fcn(l1v, l2v, theta_eta_est_err_tilt_1_vec, theta_eta_est_err_tilt_2_vec)
%%%% 固定时间跟随者期望速度分布式观测器
iiuav = 2;
d_eta_d_est_2 = -l1v * theta_eta_est_err_tilt_1_vec(:,iiuav) - l2v * theta_eta_est_err_tilt_2_vec(:,iiuav);

== matlab function sim_new_traj_only_pos_ctrl/fixed-time distributed follower desire velocity observer agent 3 ==
  data: l1v input; d_eta_d_est_3 output; l2v input; theta_eta_est_err_tilt_1_vec input; theta_eta_est_err_tilt_2_vec input
function d_eta_d_est_3 = fcn(l1v, l2v, theta_eta_est_err_tilt_1_vec, theta_eta_est_err_tilt_2_vec)
%%%% 固定时间跟随者期望速度分布式观测器
iiuav = 3;
d_eta_d_est_3 = -l1v * theta_eta_est_err_tilt_1_vec(:,iiuav) - l2v * theta_eta_est_err_tilt_2_vec(:,iiuav);

== matlab function sim_new_traj_only_pos_ctrl/fixed-time distributed follower desire velocity observer agent 4 ==
  data: l1v input; d_eta_d_est_4 output; l2v input; theta_eta_est_err_tilt_1_vec input; theta_eta_est_err_tilt_2_vec input
function d_eta_d_est_4 = fcn(l1v, l2v, theta_eta_est_err_tilt_1_vec, theta_eta_est_err_tilt_2_vec)
%%%% 固定时间跟随者期望速度分布式观测器
iiuav = 4;
d_eta_d_est_4 = -l1v * theta_eta_est_err_tilt_1_vec(:,iiuav) - l2v * theta_eta_est_err_tilt_2_vec(:,iiuav);

== matlab function sim_new_traj_only_pos_ctrl/fixed-time distributed follower desire velocity observer agent 5 ==
  data: l1v input; d_eta_d_est_5 output; l2v input; theta_eta_est_err_tilt_1_vec input; theta_eta_est_err_tilt_2_vec input
function d_eta_d_est_5 = fcn(l1v, l2v, theta_eta_est_err_tilt_1_vec, theta_eta_est_err_tilt_2_vec)
%%%% 固定时间跟随者期望速度分布式观测器
iiuav = 5;
d_eta_d_est_5 = -l1v * theta_eta_est_err_tilt_1_vec(:,iiuav) - l2v * theta_eta_est_err_tilt_2_vec(:,iiuav);

== matlab function sim_new_traj_only_pos_ctrl/trans to column41 ==
  data: x input; y output
function y = fcn(x)
y = x(:);

== matlab function sim_new_traj_only_pos_ctrl/trans to column42 ==
  data: x input; y output
function y = fcn(x)
y = x(:);

== matlab function sim_new_traj_only_pos_ctrl/trans to column43 ==
  data: x input; y output
function y = fcn(x)
y = x(:);

== matlab function sim_new_traj_only_pos_ctrl/trans to column44 ==
  data: x input; y output
function y = fcn(x)
y = x(:);

== matlab function sim_new_traj_only_pos_ctrl/cal abs 8 ==
  data: x input; y output
function y = fcn(x)
y = abs(x(:));

== matlab function sim_new_traj_only_pos_ctrl/trans to column45 ==
  data: x input; y output
function y = fcn(x)
y = x(:);

== matlab function sim_new_traj_only_pos_ctrl/trans to column46 ==
  data: x input; y output
function y = fcn(x)
y = x(:);

== matlab function sim_new_traj_only_pos_ctrl/trans to column47 ==
  data: x input; y output
function y = fcn(x)
y = x(:);

== matlab function sim_new_traj_only_pos_ctrl/trans to column48 ==
  data: x input; y output
function y = fcn(x)
y = x(:);

== matlab function sim_new_traj_only_pos_ctrl/trans to column49 ==
  data: x input; y output
function y = fcn(x)
y = x(:);

== matlab function sim_new_traj_only_pos_ctrl/trans to column50 ==
  data: x input; y output
function y = fcn(x)
y = x(:);

== matlab function sim_new_traj_only_pos_ctrl/trans to column51 ==
  data: x input; y output
function y = fcn(x)
y = x(:);

== matlab function sim_new_traj_only_pos_ctrl/trans to column52 ==
  data: x input; y output
function y = fcn(x)
y = x(:);

== matlab function sim_new_traj_only_pos_ctrl/trans to column53 ==
  data: x input; y output
function y = fcn(x)
y = x(:);

== matlab function sim_new_traj_only_pos_ctrl/trans to column54 ==
  data: x input; y output
function y = fcn(x)
y = x(:);

== matlab function sim_new_traj_only_pos_ctrl/cal theta_err_ksi agent 4 ==
  data: alfa_theta input; err_ksi_squ_1_node_4 input; theta_err_ksi_1_4 output; err_ksi_squ_2_node_4 input; err_ksi_vec input; theta_err_ksi_2_4 output
function [theta_err_ksi_1_4, theta_err_ksi_2_4] = fcn(alfa_theta, err_ksi_squ_1_node_4, err_ksi_squ_2_node_4, err_ksi_vec)
%%%% 计算平滑递增函数
iiuav = 4;
theta_err_ksi_1_4 = err_ksi_squ_1_node_4(:) .* ( -1 + 2 ./ ( 1 + exp( -alfa_theta .* err_ksi_vec(:,iiuav) ) ) );
theta_err_ksi_2_4 = err_ksi_squ_2_node_4(:) .* ( -1 + 2 ./ ( 1 + exp( -alfa_theta .* err_ksi_vec(:,iiuav) ) ) );

== matlab function sim_new_traj_only_pos_ctrl/trans to column55 ==
  data: x input; y output
function y = fcn(x)
y = x(:);

== matlab function sim_new_traj_only_pos_ctrl/trans to column56 ==
  data: x input; y output
function y = fcn(x)
y = x(:);

== matlab function sim_new_traj_only_pos_ctrl/trans to column57 ==
  data: x input; y output
function y = fcn(x)
y = x(:);

== matlab function sim_new_traj_only_pos_ctrl/trans to column58 ==
  data: x input; y output
function y = fcn(x)
y = x(:);

== matlab function sim_new_traj_only_pos_ctrl/trans to column59 ==
  data: x input; y output
function y = fcn(x)
y = x(:);

== matlab function sim_new_traj_only_pos_ctrl/trans to column60 ==
  data: x input; y output
function y = fcn(x)
y = x(:);

== matlab function sim_new_traj_only_pos_ctrl/combine formation control input ==
  data: eta_i_vec output; ksi_i_vec output; eta_1 input; eta_2 input; eta_3 input; eta_4 input; eta_5 input; ksi_1 input; ksi_2 input; ksi_3 input; ksi_4 input; ksi_5 input
function [eta_i_vec, ksi_i_vec] = fcn(eta_1, eta_2, eta_3, eta_4, eta_5, ...
                                                                ksi_1, ksi_2, ksi_3, ksi_4, ksi_5)
%%%% 合并领导者编队跟踪误差结果
eta_i_vec = [eta_1(:), eta_2(:), eta_3(:), eta_4(:), eta_5(:)];
ksi_i_vec = [ksi_1(:), ksi_2(:), ksi_3(:), ksi_4(:), ksi_5(:)];

== matlab function sim_new_traj_only_pos_ctrl/choose ksi_est_err 7 ==
  data: x input; y output
function y = fcn(x)
iiuav = 4;
y = x(:,iiuav);
